simulink model "Ex_1_Potentiometer_Position_Measurement"  (R2020a)
settings: Solver=FixedStepAuto  StartTime=0.0  StopTime=3  FixedStep=0.000001  RelTol=1e-3
values from neighbouring files (symbols this model uses):
  J = 0.005    [motor_parameters.mat]
  Ke = 2.3    [motor_parameters.mat]
  Kf = 0.3    [motor_parameters.mat]
  Kt = 2.19    [motor_parameters.mat]
  L = 1    [motor_parameters.mat]
  R = 1.1    [motor_parameters.mat]
libraries: fl_lib x3, nesl_utility x3, ee_lib x1
settings Model: Creator=alexr  LastModifiedBy=alexr

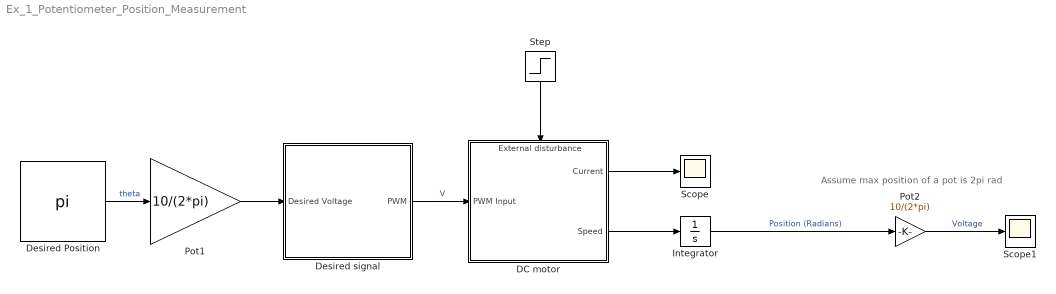
== system Ex_1_Potentiometer_Position_Measurement ==
  note: Assume max position of a pot is 2pi rad
  DC motor : Subsystem
      settings: PortSchema="{\"entries\":[{\"content\":{\"sides\":[{\"content\":{\"connectorIds\":[\"In1\"]},\"type\":\"ConnectorPlacement.EquallySpacedRectSide\",\"uuid\":\"b8964f03-f732-4eca-8bb3-271c6a142913\"},{\"content\":{\"connectorIds\":[\"Out1\",\"Out2\"],\"side\":\"RIGHT\"},\"type\":\"ConnectorPlacement.EquallySpacedRectSide\",\"uuid\":\"d9454742-672e-4fe5-95f0-bbd13d54c419\"},{\"content\":{\"connectorIds\":[\"In2\"],\"side\":\"TOP\"},\"type\":\"ConnectorPlacement.EquallySpacedRectSide\",\"uuid\":\"e6caae02-41c3-4a6e-bc88-5a1dbae17927\"}]},\"type\":\"ConnectorPlacement.EquallySpacedConnector\",\"uuid\":\"63b5fd96-b4f9-40de-b12b-448e4637e2c5\"}],\"packageUris\":[\"http://schema.mathworks.com/mf0/Connector/19700101\"],\"version\":\"1.0\"}"
  Desired Position : Constant  Value=pi
  Desired signal : Subsystem
  Integrator : Integrator
  Pot1 : Gain  Gain=10/(2*pi)
  Pot2 : Gain  Gain=10/(2*pi)
  Scope : Scope
  Scope1 : Scope
  "Step " : Step  Time=0.5  After=0  SampleTime=0
  wires:
  DC motor/2(Speed) -> Integrator/1
  "Step "/1 -> DC motor/2(External disturbance)
  DC motor/1(Current) -> Scope/1
  Integrator/1 -> Pot2/1  "Position (Radians)"
  Pot2/1 -> Scope1/1  "Voltage"
  Pot1/1 -> Desired signal/1(Desired Voltage)
  Desired signal/1(PWM) -> DC motor/1(PWM Input)  "V"
  Desired Position/1 -> Pot1/1  "theta"

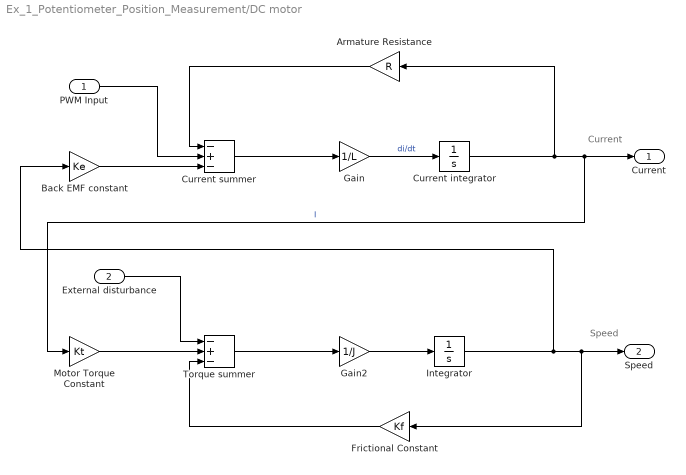
== system Ex_1_Potentiometer_Position_Measurement/DC motor ==
  note: Speed
  note: Current
  PWM Input : Inport
  External disturbance : Inport  Port=2
  Armature Resistance : Gain  Gain=R
  Back EMF constant : Gain  Gain=Ke
  Current integrator : Integrator
  Current summer : Sum  Inputs=-+-
  Frictional Constant : Gain  Gain=Kf
  Gain : Gain  Gain=1/L
  Gain2 : Gain  Gain=1/J
  Integrator : Integrator
  Motor Torque Constant : Gain  Gain=Kt
  Torque summer : Sum  Inputs=-+-
  Current : Outport
  Speed : Outport  Port=2
  wires:
  Current summer/1 -> Gain/1
  Gain2/1 -> Integrator/1
  Integrator/1 -> Back EMF constant/1, Speed/1, Frictional Constant/1
  Torque summer/1 -> Gain2/1
  Armature Resistance/1 -> Current summer/1
  PWM Input/1 -> Current summer/2
  Gain/1 -> Current integrator/1  "di/dt"
  Motor Torque Constant/1 -> Torque summer/2
  External disturbance/1 -> Torque summer/1
  Frictional Constant/1 -> Torque summer/3
  Current integrator/1 -> Armature Resistance/1, Current/1, Motor Torque Constant/1  "I"
  Back EMF constant/1 -> Current summer/3

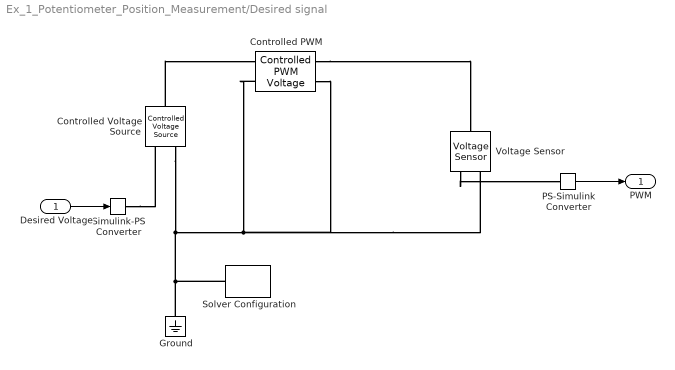
== system Ex_1_Potentiometer_Position_Measurement/Desired signal ==
  Desired Voltage : Inport
  "Controlled PWM " : ee_lib/Integrated Circuits/Controlled PWM Voltage  F=4000 Hz  TD=0 s  pulse_width_offset=0 s  pulse_min=0 s  Vmin=0 V  Vmax=10 V  Vm=10 V  pwm_or_av=2  event_type=1  sample_time=1e-6 s  u_min=0  u_max=5
  Controlled Voltage Source : fl_lib/Electrical/Electrical Sources/Controlled Voltage Source
  "Ground " : fl_lib/Electrical/Electrical Elements/Electrical Reference
      settings: SourceProductBaseCode=MT,SS
  PS-Simulink Converter : nesl_utility/PS-Simulink Converter  PhysicalDomain=network_engine_domain  SubClassName=ps_output  LeftPortType=input  RightPortType=output  PseudoPeriodic=off  Frequencies=[]  Unit=inherit  AffineConversion=off
  Simulink-PS Converter : nesl_utility/Simulink-PS Converter  PhysicalDomain=network_engine_domain  SubClassName=ps_input  LeftPortType=input  RightPortType=output  PseudoPeriodic=off  Frequencies=[]  NoiseDistribution=none  NoiseParameters=[]  Unit=1  AffineConversion=off  FilteringAndDerivatives=provide  SimscapeFilterOrder=1  InputFilterTimeConstant=0.001  UdotUserProvided=0
  "Solver Configuration " : nesl_utility/Solver Configuration  PhysicalDomain=network_engine_domain  SubClassName=solver  LeftPortType=input  RightPortType=generic  Tones=[]  Harmonics=[]  SimulateNoise=off  Profile=off  UseLocalSampling=off  EnableSwitchedLinearOptims=on  FrequencyDomain=off  UseCCode=off  RelTol=0.001  AbsTol=1e-06  MinStep=1e-09  ToWorkspace=off  RevertToSquareIcSolve=off  NumHomotopyIterations=100  PhasorMode=off  PhasorModeNumHarmonics=1  DoDC=off  ResidualTolerance=1e-09  UseLocalSolver=off  LocalSolverChoice=NE_BACKWARD_EULER_ADVANCER  LocalSolverSampleTime=0.001  DoFixedCost=off  MaxNonlinIter=3  MaxModeIter=2  LinearAlgebra=auto  EquationFormulation=NE_TIME_EF  DelaysMemoryBudget=1024  AutomaticFiltering=on  FilteringTimeConstant=0.001  PartitionStorageMethod=AS_NEEDED  PartitionMemoryBudget=1024  PartitionMethod=ROBUST
  Voltage Sensor : fl_lib/Electrical/Electrical Sensors/Voltage Sensor
  PWM : Outport
  wires:
  PS-Simulink Converter/1 -> PWM/1
  Desired Voltage/1 -> Simulink-PS Converter/1
  connections:
  "Solver Configuration "/RConn1 -- Voltage Sensor/RConn2 -- "Controlled PWM "/RConn2 -- "Controlled PWM "/LConn2 -- Controlled Voltage Source/RConn2 -- "Ground "/LConn1
  "Controlled PWM "/RConn1 -- Voltage Sensor/LConn1
  Voltage Sensor/RConn1 -- PS-Simulink Converter/LConn1
  Controlled Voltage Source/LConn1 -- "Controlled PWM "/LConn1
  Simulink-PS Converter/RConn1 -- Controlled Voltage Source/RConn1
